simulink model "ad_configmodel"  (R2015b)
settings: Solver=FixedStepDiscrete  SolverMode=SingleTasking  StartTime=0.0  StopTime=SimEnd+Ts2*NTaps*2  RelTol=1e-3
PreLoadFcn:
  | Param_fir
values from neighbouring files (symbols this model uses):
  Fpass = 20    [Param_fir.m]
  Fs = 100    [Param_fir.m]
  NTaps = 128    [Param_fir.m]
  Numerator = firls(NTaps-1, [0 Fpass Fstop Fs/2]/(Fs/2), [1 1 0 0], [Wpass Wstop])    [Param_fir.m]
  SimEnd = 0.0025    [Param_fir.m]
  Ts1 = Ts2/NTaps    (= 7.8125e-05)    [Param_fir.m]
  Ts2 = 1/Fs    (= 0.01)    [Param_fir.m]
undefined symbols (not defined in the file or in its folder): dfilt
libraries: dspsrcs4 x2, dspobslib x1, ad_configsub x1, hdlsllib x1, simulink x1
Description:
  | RAM-based FIR Filter
  | This model shows how to use Simulink(R) HDL Coder(TM) to generate and verify HDL code for a RAM-based FIR filter using a multiply-accumulate architecture.
settings Model: Creator=bogilvie  LastModifiedBy=amatsumo
settings DataIOCC: SaveFormat=Array  SignalLoggingSaveFormat=ModelDataLogs  SaveOutput=off  SignalLogging=off  SaveTime=off
settings OptimizationCC: BlockReduction=off  ConditionallyExecuteInputs=off  DefaultParameterBehavior=Inlined  ExpressionDepthLimit=2147483647  InitFltsAndDblsToZero=on
settings DebuggingCC: AlgebraicLoopMsg=error  UnderspecifiedInitializationDetection=Classic  MergeDetectMultiDrivingBlocksExec=none  SignalResolutionControl=TryResolveAllWithWarning  SolverPrmCheckMsg=warning  SingleTaskRateTransMsg=error  IntegerOverflowMsg=none  ParameterOverflowMsg=warning  ParameterPrecisionLossMsg=none  FcnCallInpInsideContextMsg=UseLocalSettings  StateNameClashWarn=warning  IntegerSaturationMsg=none
settings HardwareCC: ProdBitPerPointer=32  ProdLargestAtomicFloat=None  ProdIntDivRoundTo=Undefined  ProdEndianess=Unspecified  ProdWordSize=32  ProdHWDeviceType=ASIC/FPGA->ASIC/FPGA  ProdEqTarget=off
settings SFSimCC: SFSimEcho=off
settings GRTTargetCC: GeneratePreprocessorConditionals=Disable all  CombineOutputUpdateFcns=off  GRTInterface=on
settings ConfigComp: CovModelRefEnable=Off  CovSFcnEnable=off

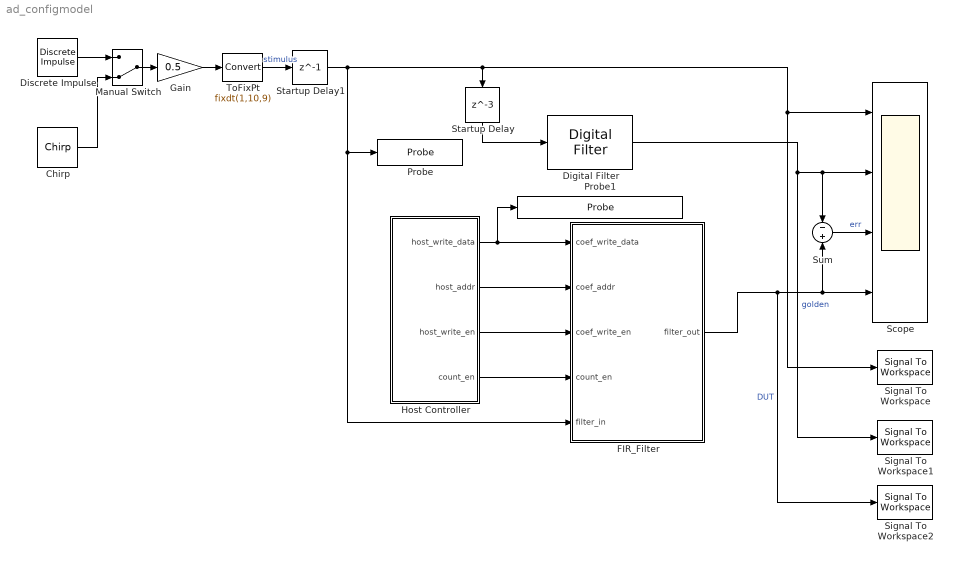
== system ad_configmodel ==
  Chirp : dspsrcs4/Chirp  sweep=Linear  mode=Unidirectional  f0=Fpass/100  f1=Fs/2  t1=SimEnd+Ts2*NTaps*2  Tsweep=SimEnd+Ts2*NTaps*2  phase=0  Ts=Ts2  spf=1  datatype=Double  OutputFrames=on
  Digital Filter : dspobslib/Digital Filter  TypePopup=FIR (all zeros)  IIRFiltStruct=Direct form II transposed  AllPoleFiltStruct=Direct form  FIRFiltStruct=Direct form  CoeffSource=Specify via dialog  NumCoeffs=Numerator  DenCoeffs=[1 0.1]  BiQuadCoeffs=[1 0.3 0.4 1 0.1 0.2]  LatticeCoeffs=[0.2 0.4]  denIgnore=on  FiltPerSampPopup=One filter per frame  IC=0  ICnum=0  ICden=0  firstCoeffMode=Binary point scaling  firstCoeffWordLength=16  firstCoeffFracLength=15  accumMode=Binary point scaling  accumWordLength=30  accumFracLength=24  prodOutputMode=Binary point scaling  prodOutputWordLength=26  prodOutputFracLength=24  roundingMode=Floor  overflowMode=off  ScaleValues=1  scaleValueFracLength=14  stageInFracLength=15  stageOutFracLength=15  FilterSource=Specify via dialog  dfiltObjectName=dfilt.dffir([1 2 1])
  Discrete Impulse : dspsrcs4/Discrete  Impulse  Delay=10  SampleTime=Ts2  FrameSample=1  OutputFrames=on  dataType=double  isSigned=on  wordLen=16  udDataType=sfix(16)  fracBitsMode=Best precision  numFracBits=15  OutDataTypeStr=double  LastOutDataTypeStr=double
  FIR_Filter : Subsystem
  Gain : Gain  Gain=0.5
  Host Controller : Subsystem
  Manual Switch : ManualSwitch  CurrentSetting=0
  Probe : Probe  ProbeWidth=off  ProbeComplexSignal=off
  Probe1 : Probe  ProbeWidth=off  ProbeComplexSignal=off
  Scope : Scope  NumInputPorts=4
  Signal To Workspace : SignalToWorkspace  VariableName=filter_in
      settings: CopyFcn=dspblkcopystw(gcbh);  Save2DSignal=3-D array (concatenate along third dimension)
  Signal To Workspace1 : SignalToWorkspace  VariableName=filter_out
      settings: CopyFcn=dspblkcopystw(gcbh);  Save2DSignal=3-D array (concatenate along third dimension)
  Signal To Workspace2 : SignalToWorkspace  VariableName=dut_out
      settings: CopyFcn=dspblkcopystw(gcbh);  Save2DSignal=3-D array (concatenate along third dimension)
  Startup Delay : Delay  DelayLength=3  InputProcessing=Inherited
  Startup Delay1 : Delay  DelayLength=1  InputProcessing=Inherited
  Sum : Sum  Inputs=-|+
  ToFixPt : DataTypeConversion  OutDataTypeStr=fixdt(1,10,9)  RndMeth=Nearest  SaturateOnIntegerOverflow=on
  wires:
  ToFixPt/1 -> Startup Delay1/1  "stimulus"
  Digital Filter/1 -> Sum/1, Scope/2, Signal To Workspace1/1  "golden"
  FIR_Filter/1(filter_out) -> Scope/4, Sum/2, Signal To Workspace2/1  "DUT"
  Startup Delay/1 -> Digital Filter/1
  Manual Switch/1 -> Gain/1
  Discrete Impulse/1 -> Manual Switch/1
  Chirp/1 -> Manual Switch/2
  Gain/1 -> ToFixPt/1
  Sum/1 -> Scope/3  "err"
  Startup Delay1/1 -> Startup Delay/1, Scope/1, Signal To Workspace/1, FIR_Filter/5(filter_in), Probe/1
  Host Controller/1(host_write_data) -> FIR_Filter/1(coef_write_data), Probe1/1
  Host Controller/2(host_addr) -> FIR_Filter/2(coef_addr)
  Host Controller/3(host_write_en) -> FIR_Filter/3(coef_write_en)
  Host Controller/4(count_en) -> FIR_Filter/4(count_en)

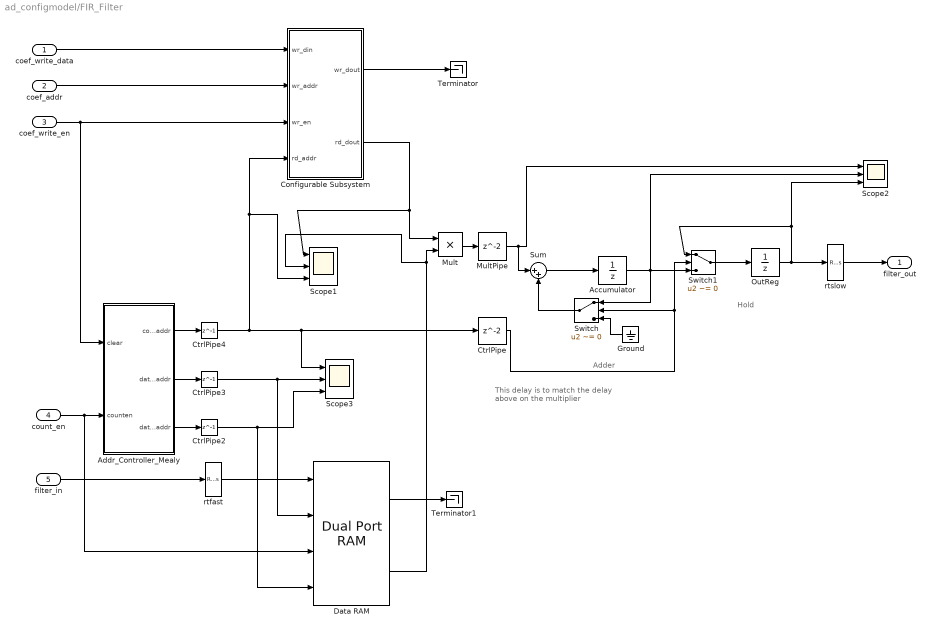
== system ad_configmodel/FIR_Filter ==
  note: This delay is to match the
      | delay above on the multiplier
  note: Hold
  note: Adder
  coef_write_data : Inport  PortDimensions=1
  coef_addr : Inport  Port=2
  coef_write_en : Inport  Port=3  OutDataTypeStr=boolean
  count_en : Inport  Port=4  OutDataTypeStr=boolean
  filter_in : Inport  Port=5  PortDimensions=1
  Accumulator : UnitDelay  SampleTime=-1
  Addr_Controller_Mealy : Stateflow chart  TreatAsAtomicUnit=on
  Configurable Subsystem : Subsystem  BlockChoice=ConfigSubLUT
      settings: AttributesFormatString=%<BlockChoice>  MemberBlocks=ConfigSubLUT,ConfigSubRAM
      settings: TemplateBlock=|
      | ad_configsub/Configurable
      | Subsystem
  CtrlPipe : Delay  InputProcessing=Inherited
  CtrlPipe2 : Delay  DelayLength=1  InputProcessing=Inherited
  CtrlPipe3 : Delay  DelayLength=1  InputProcessing=Inherited
  CtrlPipe4 : Delay  DelayLength=1  InputProcessing=Inherited
  Data RAM : hdlsllib/HDL Operations/Dual Port RAM  ram_size=ceil(log2(NTaps))
  Ground : Ground
  Mult : Product
  MultPipe : Delay  InputProcessing=Inherited
  OutReg : UnitDelay  SampleTime=Ts1
  Scope1 : Scope  NumInputPorts=3
  Scope2 : Scope  NumInputPorts=3
  Scope3 : Scope  NumInputPorts=3
  Sum : Sum  Inputs=|++  OutDataTypeStr=fixdt(1,30,24)
  Switch : Switch  Criteria=u2 ~= 0
  Switch1 : Switch  Criteria=u2 ~= 0
  Terminator : Terminator
  Terminator1 : Terminator
  rtfast : RateTransition
  rtslow : RateTransition  OutPortSampleTime=Ts2
  filter_out : Outport
  wires:
  coef_addr/1 -> Configurable Subsystem/2(wr_addr)
  coef_write_en/1 -> Configurable Subsystem/3(wr_en), Addr_Controller_Mealy/1(clear)
  Addr_Controller_Mealy/1(coef_rdaddr) -> CtrlPipe4/1
  Data RAM/2 -> Mult/2, Scope1/2
  Mult/1 -> MultPipe/1
  Sum/1 -> Accumulator/1
  Switch/1 -> Sum/2
  Accumulator/1 -> Switch/1, Switch1/3, Scope2/2
  count_en/1 -> Data RAM/3, Addr_Controller_Mealy/2(counten)
  Ground/1 -> Switch/3
  rtslow/1 -> filter_out/1
  MultPipe/1 -> Sum/1, Scope2/1
  OutReg/1 -> rtslow/1, Switch1/1, Scope2/3
  Switch1/1 -> OutReg/1
  filter_in/1 -> rtfast/1
  rtfast/1 -> Data RAM/1
  CtrlPipe/1 -> Switch/2, Switch1/2
  Configurable Subsystem/1(wr_dout) -> Terminator/1
  Addr_Controller_Mealy/2(data_wraddr) -> CtrlPipe3/1
  Addr_Controller_Mealy/3(data_rdaddr) -> CtrlPipe2/1
  CtrlPipe2/1 -> Data RAM/4, Scope3/3
  CtrlPipe3/1 -> Data RAM/2, Scope3/2
  CtrlPipe4/1 -> Configurable Subsystem/4(rd_addr), Scope1/3, CtrlPipe/1, Scope3/1
  Data RAM/1 -> Terminator1/1
  coef_write_data/1 -> Configurable Subsystem/1(wr_din)
  Configurable Subsystem/2(rd_dout) -> Mult/1, Scope1/1

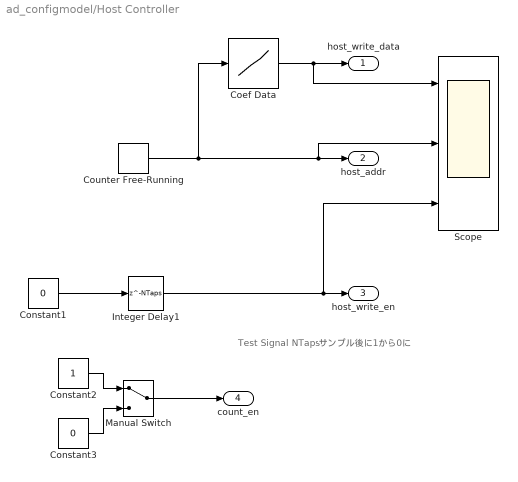
== system ad_configmodel/Host Controller ==
  note: Test Signal
      | NTapsサンプル後に1から0に
  Coef Data : Lookup_n-D  NumberOfTableDimensions=1  BreakpointsForDimension1=[0:NTaps-1]  IndexSearchMethod=Evenly spaced points  Table=fliplr(Numerator)  ExtrapMethod=Clip  OutDataTypeStr=fixdt(1,16,15)  InputSameDT=on
  Constant1 : Constant  Value=0  OutDataTypeStr=boolean
  Constant2 : Constant  OutDataTypeStr=boolean
  Constant3 : Constant  Value=0  OutDataTypeStr=boolean
  Counter Free-Running : simulink/Sources/Counter Free-Running  NumBits=ceil(log2(NTaps))  tsamp=-1
  Integer Delay1 : Delay  DelayLength=NTaps  InitialCondition=1  InputProcessing=Inherited
  Manual Switch : ManualSwitch
  Scope : Scope  NumInputPorts=3
  host_write_data : Outport
  host_addr : Outport  Port=2
  host_write_en : Outport  Port=3
  count_en : Outport  Port=4
  wires:
  Counter Free-Running/1 -> Coef Data/1, host_addr/1, Scope/2
  Coef Data/1 -> host_write_data/1, Scope/1
  Integer Delay1/1 -> host_write_en/1, Scope/3
  Manual Switch/1 -> count_en/1
  Constant1/1 -> Integer Delay1/1
  Constant2/1 -> Manual Switch/1
  Constant3/1 -> Manual Switch/2

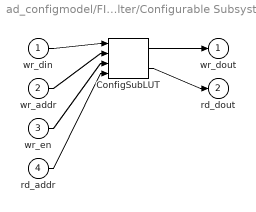
== system ad_configmodel/FIR_Filter/Configurable Subsystem ==
  wr_din : Inport
  wr_addr : Inport  Port=2
  wr_en : Inport  Port=3
  rd_addr : Inport  Port=4
  ConfigSubLUT : ad_configsub/ConfigSubLUT
  wr_dout : Outport
  rd_dout : Outport  Port=2
  wires:
  wr_din/1 -> ConfigSubLUT/1
  wr_addr/1 -> ConfigSubLUT/2
  wr_en/1 -> ConfigSubLUT/3
  rd_addr/1 -> ConfigSubLUT/4
  ConfigSubLUT/1 -> wr_dout/1
  ConfigSubLUT/2 -> rd_dout/1

== stateflow chart ad_configmodel/FIR_Filter/Addr_Controller_Mealy ==
  settings: updateMethod=DISCRETE  stateMachineType=MEALY_MACHINE  executeAtInitialization=1  initializeOutput=1
  state Increment1/
  state Init/
  state increment_action [function]
    (default) -> (junction 97) : {
        | Addr_coefrd++;
        | }
    (junction 97) -> (junction 101) [order 1] : [Addr_datawr>=Addr_coefrd]{
        | Addr_datard=Addr_datawr-Addr_coefrd;
        | }
    (junction 97) -> (junction 99) [order 2] : {
        | Addr_datard=Addr_datawr+NTaps-Addr_coefrd;
        | }
  state init_action [function]
    (default) -> (junction 61) : {
        | Addr_coefrd=0;
        | }
        | /*
        | 係数アドレスリセット
        | */
    (junction 61) -> (junction 83) [order 1] : [Addr_datawr>=NTaps-1]
        | {
        | Addr_datawr=0;
        | Addr_datard=0;
        | }
        | /*
        | Dataアドレスリセット
        | */
    (junction 61) -> (junction 85) [order 2] : {
        | Addr_datawr++;
        | Addr_datard=Addr_datawr;
        | }
  state output_action [function]
    (default) -> (junction 69) : {
        | coef_rdaddr=Addr_coefrd;
        | data_rdaddr=Addr_datard;
        | data_wraddr=Addr_datawr;
        | }
  state Nop/
  (default) -> Init
  (junction 110) -> Increment1 [order 1] : [counten==1]
      | {
      | increment_action();
      | output_action();
      | }
  Increment1 -> Increment1 [order 1] : [clear==0&&counten==1&&Addr_coefrd<NTaps-1]{
      | increment_action();
      | output_action();
      | }
  Init -> (junction 110) [order 1] : [clear==0]
  (junction 110) -> Nop [order 2] : {
      | output_action();
      | }
  Increment1 -> Init [order 3] : /*
      | [clear==1||Addr_coefrd>=NTaps-1]
      | */
      | {
      | init_action();
      | output_action();
      | }
  Nop -> Increment1 [order 1] : /*[clear==0&&counten==1&&Addr_coefrd<NTaps-1]*/
      | [clear==0&&counten==1]
      | {
      | increment_action();
      | output_action();
      | }
  Increment1 -> Nop [order 2] : [counten==0]{
      | output_action();
      | }
  Init -> Init [order 2] : {
      | output_action();
      | }
  Nop -> Init [order 2] : [clear==1]{
      | init_action();
      | output_action();
      | }
  Nop -> Nop [order 3] : {
      | output_action();
      | }
  data: clear input boolean; counten input boolean; coef_rdaddr output fixdt(0,ceil(log2(NTaps)),0); data_wraddr output fixdt(0,ceil(log2(NTaps)),0); data_rdaddr output fixdt(0,ceil(log2(NTaps)),0); Addr_coefrd local uint8; Addr_datard local uint8; Addr_datawr local uint8; NTaps parameter uint8
